simulink model "case7"  (R2024b)
settings: Solver=FixedStepAuto  StartTime=0  StopTime=1  FixedStep=1e-7  RelTol=1e-3
values from neighbouring files (symbols this model uses):
  SG_D_1_D = 0.01056    [IEEE9_case_parameters.m]    (also in case1_parameters.m; case2_parameters.m; case3_parameters.m; case4_parameters.m)
  SG_D_1_EnableSaturation = 0    [IEEE9_case_parameters.m]    (also in case1_parameters.m; case2_parameters.m; case3_parameters.m; case4_parameters.m)
  SG_D_1_f0 = 60    [IEEE9_case_parameters.m]    (also in case1_parameters.m; case2_parameters.m; case3_parameters.m; case4_parameters.m)
  SG_D_1_H = 7.5    [IEEE9_case_parameters.m]    (also in case1_parameters.m; case2_parameters.m; case3_parameters.m; case4_parameters.m)
  SG_D_1_K_A = 20    [IEEE9_case_parameters.m]    (also in case1_parameters.m; case2_parameters.m; case3_parameters.m; case4_parameters.m)
  SG_D_1_K_E = 1.000000e+1    (= 10)    [IEEE9_case_parameters.m]    (also in case1_parameters.m; case2_parameters.m; case3_parameters.m; case4_parameters.m)
  SG_D_1_K_F = 2.363    [IEEE9_case_parameters.m]    (also in case1_parameters.m; case2_parameters.m; case3_parameters.m; case4_parameters.m)
  SG_D_1_K_s = 0.5    [IEEE9_case_parameters.m]    (also in case1_parameters.m = 5; case2_parameters.m = 5; case3_parameters.m = 5; case4_parameters.m = 5)
  SG_D_1_R_a = 0.001088    [IEEE9_case_parameters.m]    (also in case1_parameters.m; case2_parameters.m; case3_parameters.m; case4_parameters.m)
  SG_D_1_S_A = 1    [IEEE9_case_parameters.m]    (also in case1_parameters.m; case2_parameters.m; case3_parameters.m; case4_parameters.m)
  SG_D_1_S_B = 0.103    [IEEE9_case_parameters.m]    (also in case1_parameters.m; case2_parameters.m; case3_parameters.m; case4_parameters.m)
  SG_D_1_S_N = 10.659857    [IEEE9_case_parameters.m]    (also in case1_parameters.m; case2_parameters.m; case3_parameters.m; case4_parameters.m)
  SG_D_1_SpeedPara = 200    [IEEE9_case_parameters.m]    (also in case1_parameters.m; case2_parameters.m; case3_parameters.m; case4_parameters.m)
  SG_D_1_T_0 = 0.720173    [IEEE9_case_parameters.m]    (also in case1_parameters.m = 0.755522; case2_parameters.m = 0.808931; case3_parameters.m = 0.869402; case4_parameters.m = 0.729316)
  SG_D_1_T_1 = 0.3    [IEEE9_case_parameters.m]    (also in case1_parameters.m; case2_parameters.m; case3_parameters.m; case4_parameters.m)
  SG_D_1_T_2 = 0.05    [IEEE9_case_parameters.m]    (also in case1_parameters.m; case2_parameters.m; case3_parameters.m; case4_parameters.m)
  SG_D_1_T_3 = 0.02    [IEEE9_case_parameters.m]    (also in case1_parameters.m; case2_parameters.m; case3_parameters.m; case4_parameters.m)
  SG_D_1_T_4 = 0.005    [IEEE9_case_parameters.m]    (also in case1_parameters.m; case2_parameters.m; case3_parameters.m; case4_parameters.m)
  SG_D_1_T_A = 0.02    [IEEE9_case_parameters.m]    (also in case1_parameters.m; case2_parameters.m; case3_parameters.m; case4_parameters.m)
  SG_D_1_T_dd = 8.000000e+0    (= 8)    [IEEE9_case_parameters.m]    (also in case1_parameters.m; case2_parameters.m; case3_parameters.m; case4_parameters.m)
  SG_D_1_T_ddd = 0.04    [IEEE9_case_parameters.m]    (also in case1_parameters.m; case2_parameters.m; case3_parameters.m; case4_parameters.m)
  SG_D_1_T_E = 0.314    [IEEE9_case_parameters.m]    (also in case1_parameters.m; case2_parameters.m; case3_parameters.m; case4_parameters.m)
  SG_D_1_T_F = 0.35    [IEEE9_case_parameters.m]    (also in case1_parameters.m; case2_parameters.m; case3_parameters.m; case4_parameters.m)
  SG_D_1_T_qd = 0.8    [IEEE9_case_parameters.m]    (also in case1_parameters.m; case2_parameters.m; case3_parameters.m; case4_parameters.m)
  SG_D_1_T_qdd = 0.02    [IEEE9_case_parameters.m]    (also in case1_parameters.m; case2_parameters.m; case3_parameters.m; case4_parameters.m)
  SG_D_1_T_speed = 0.1    [IEEE9_case_parameters.m]    (also in case1_parameters.m = 200; case2_parameters.m = 200; case3_parameters.m = 200; case4_parameters.m = 200)
  SG_D_1_T_w = 0.5    [IEEE9_case_parameters.m]    (also in case1_parameters.m; case2_parameters.m; case3_parameters.m; case4_parameters.m)
  SG_D_1_V_ref = 1.990276    [IEEE9_case_parameters.m]    (also in case1_parameters.m = 2.042296; case2_parameters.m = 2.051388; case3_parameters.m = 2.089584; case4_parameters.m = 2.01845)
  SG_D_1_w_ref = 376.991118    [IEEE9_case_parameters.m]    (also in case1_parameters.m; case2_parameters.m; case3_parameters.m; case4_parameters.m)
  SG_D_1_wb = 6.000000e+1    (= 60)    [IEEE9_case_parameters.m]    (also in case1_parameters.m; case2_parameters.m; case3_parameters.m; case4_parameters.m)
  SG_D_1_x_d = 1.9    [IEEE9_case_parameters.m]    (also in case1_parameters.m; case2_parameters.m; case3_parameters.m; case4_parameters.m)
  SG_D_1_x_dd = 0.302    [IEEE9_case_parameters.m]    (also in case1_parameters.m; case2_parameters.m; case3_parameters.m; case4_parameters.m)
  SG_D_1_x_ddd = 0.204    [IEEE9_case_parameters.m]    (also in case1_parameters.m; case2_parameters.m; case3_parameters.m; case4_parameters.m)
  SG_D_1_x_l = 0.05    [IEEE9_case_parameters.m]    (also in case1_parameters.m; case2_parameters.m; case3_parameters.m; case4_parameters.m)
  SG_D_1_x_q = 1.3    [IEEE9_case_parameters.m]    (also in case1_parameters.m; case2_parameters.m; case3_parameters.m; case4_parameters.m)
  SG_D_1_x_qd = 0.5    [IEEE9_case_parameters.m]    (also in case1_parameters.m; case2_parameters.m; case3_parameters.m; case4_parameters.m)
  SG_D_1_x_qdd = 0.3    [IEEE9_case_parameters.m]    (also in case1_parameters.m; case2_parameters.m; case3_parameters.m; case4_parameters.m)
  SG_D_2_D = 0.02    [IEEE9_case_parameters.m]    (also in case1_parameters.m; case2_parameters.m; case3_parameters.m; case4_parameters.m)
  SG_D_2_EnableSaturation = 0    [IEEE9_case_parameters.m]    (also in case1_parameters.m; case2_parameters.m; case3_parameters.m; case4_parameters.m)
  SG_D_2_f0 = 60    [IEEE9_case_parameters.m]    (also in case1_parameters.m; case2_parameters.m; case3_parameters.m; case4_parameters.m)
  SG_D_2_H = 8.000000e+0    (= 8)    [IEEE9_case_parameters.m]    (also in case1_parameters.m; case2_parameters.m; case3_parameters.m; case4_parameters.m)
  SG_D_2_K_A = 20    [IEEE9_case_parameters.m]    (also in case1_parameters.m; case2_parameters.m; case3_parameters.m; case4_parameters.m)
  SG_D_2_K_E = 1.000000e+1    (= 10)    [IEEE9_case_parameters.m]    (also in case1_parameters.m; case2_parameters.m; case3_parameters.m; case4_parameters.m)
  SG_D_2_K_F = 2.363    [IEEE9_case_parameters.m]    (also in case1_parameters.m; case2_parameters.m; case3_parameters.m; case4_parameters.m)
  SG_D_2_K_s = 0.5    [IEEE9_case_parameters.m]    (also in case1_parameters.m = 4; case2_parameters.m = 4; case3_parameters.m = 4; case4_parameters.m = 4)
  SG_D_2_R_a = 0.001088    [IEEE9_case_parameters.m]    (also in case1_parameters.m; case2_parameters.m; case3_parameters.m; case4_parameters.m)
  SG_D_2_S_A = 1    [IEEE9_case_parameters.m]    (also in case1_parameters.m; case2_parameters.m; case3_parameters.m; case4_parameters.m)
  SG_D_2_S_B = 0.103    [IEEE9_case_parameters.m]    (also in case1_parameters.m; case2_parameters.m; case3_parameters.m; case4_parameters.m)
  SG_D_2_S_N = 10.659857    [IEEE9_case_parameters.m]    (also in case1_parameters.m; case2_parameters.m; case3_parameters.m; case4_parameters.m)
  SG_D_2_SpeedPara = 200    [IEEE9_case_parameters.m]    (also in case1_parameters.m; case2_parameters.m; case3_parameters.m; case4_parameters.m)
  SG_D_2_T_0 = 1.632913    [IEEE9_case_parameters.m]    (also in case1_parameters.m = 1.632925; case2_parameters.m = 1.632915; case3_parameters.m = 1.632914; case4_parameters.m = 1.632927)
  SG_D_2_T_1 = 0.2    [IEEE9_case_parameters.m]    (also in case1_parameters.m; case2_parameters.m; case3_parameters.m; case4_parameters.m)
  SG_D_2_T_2 = 0.05    [IEEE9_case_parameters.m]    (also in case1_parameters.m; case2_parameters.m; case3_parameters.m; case4_parameters.m)
  SG_D_2_T_3 = 0.02    [IEEE9_case_parameters.m]    (also in case1_parameters.m; case2_parameters.m; case3_parameters.m; case4_parameters.m)
  SG_D_2_T_4 = 0.005    [IEEE9_case_parameters.m]    (also in case1_parameters.m; case2_parameters.m; case3_parameters.m; case4_parameters.m)
  SG_D_2_T_A = 0.02    [IEEE9_case_parameters.m]    (also in case1_parameters.m; case2_parameters.m; case3_parameters.m; case4_parameters.m)
  SG_D_2_T_dd = 7.9    [IEEE9_case_parameters.m]    (also in case1_parameters.m; case2_parameters.m; case3_parameters.m; case4_parameters.m)
  SG_D_2_T_ddd = 0.04    [IEEE9_case_parameters.m]    (also in case1_parameters.m; case2_parameters.m; case3_parameters.m; case4_parameters.m)
  SG_D_2_T_E = 0.314    [IEEE9_case_parameters.m]    (also in case1_parameters.m; case2_parameters.m; case3_parameters.m; case4_parameters.m)
  SG_D_2_T_F = 0.35    [IEEE9_case_parameters.m]    (also in case1_parameters.m; case2_parameters.m; case3_parameters.m; case4_parameters.m)
  SG_D_2_T_qd = 0.8    [IEEE9_case_parameters.m]    (also in case1_parameters.m; case2_parameters.m; case3_parameters.m; case4_parameters.m)
  SG_D_2_T_qdd = 0.015    [IEEE9_case_parameters.m]    (also in case1_parameters.m; case2_parameters.m; case3_parameters.m; case4_parameters.m)
  SG_D_2_T_speed = 0.1    [IEEE9_case_parameters.m]    (also in case1_parameters.m = 150; case2_parameters.m = 150; case3_parameters.m = 150; case4_parameters.m = 150)
  SG_D_2_T_w = 0.35    [IEEE9_case_parameters.m]    (also in case1_parameters.m; case2_parameters.m; case3_parameters.m; case4_parameters.m)
  SG_D_2_V_ref = 2.58547    [IEEE9_case_parameters.m]    (also in case1_parameters.m = 2.597896; case2_parameters.m = 2.587136; case3_parameters.m = 2.586042; case4_parameters.m = 2.599679)
  SG_D_2_w_ref = 376.991118    [IEEE9_case_parameters.m]    (also in case1_parameters.m; case2_parameters.m; case3_parameters.m; case4_parameters.m)
  SG_D_2_wb = 6.000000e+1    (= 60)    [IEEE9_case_parameters.m]    (also in case1_parameters.m; case2_parameters.m; case3_parameters.m; case4_parameters.m)
  SG_D_2_x_d = 1.8    [IEEE9_case_parameters.m]    (also in case1_parameters.m; case2_parameters.m; case3_parameters.m; case4_parameters.m)
  SG_D_2_x_dd = 0.302    [IEEE9_case_parameters.m]    (also in case1_parameters.m; case2_parameters.m; case3_parameters.m; case4_parameters.m)
  SG_D_2_x_ddd = 0.204    [IEEE9_case_parameters.m]    (also in case1_parameters.m; case2_parameters.m; case3_parameters.m; case4_parameters.m)
  SG_D_2_x_l = 0.05    [IEEE9_case_parameters.m]    (also in case1_parameters.m; case2_parameters.m; case3_parameters.m; case4_parameters.m)
  SG_D_2_x_q = 1.25    [IEEE9_case_parameters.m]    (also in case1_parameters.m; case2_parameters.m; case3_parameters.m; case4_parameters.m)
  SG_D_2_x_qd = 0.5    [IEEE9_case_parameters.m]    (also in case1_parameters.m; case2_parameters.m; case3_parameters.m; case4_parameters.m)
  SG_D_2_x_qdd = 0.3    [IEEE9_case_parameters.m]    (also in case1_parameters.m; case2_parameters.m; case3_parameters.m; case4_parameters.m)
  SG_D_3_D = 0.02    [IEEE9_case_parameters.m]    (also in case1_parameters.m; case2_parameters.m; case3_parameters.m; case4_parameters.m)
  SG_D_3_EnableSaturation = 0    [IEEE9_case_parameters.m]    (also in case1_parameters.m; case2_parameters.m; case3_parameters.m; case4_parameters.m)
  SG_D_3_f0 = 60    [IEEE9_case_parameters.m]    (also in case1_parameters.m; case2_parameters.m; case3_parameters.m; case4_parameters.m)
  SG_D_3_H = 7.7    [IEEE9_case_parameters.m]    (also in case1_parameters.m; case2_parameters.m; case3_parameters.m; case4_parameters.m)
  SG_D_3_K_A = 20    [IEEE9_case_parameters.m]    (also in case1_parameters.m; case2_parameters.m; case3_parameters.m; case4_parameters.m)
  SG_D_3_K_E = 1.000000e+1    (= 10)    [IEEE9_case_parameters.m]    (also in case1_parameters.m; case2_parameters.m; case3_parameters.m; case4_parameters.m)
  SG_D_3_K_F = 2.363    [IEEE9_case_parameters.m]    (also in case1_parameters.m; case2_parameters.m; case3_parameters.m; case4_parameters.m)
  SG_D_3_K_s = 0.2    [IEEE9_case_parameters.m]    (also in case1_parameters.m = 2; case2_parameters.m = 2; case3_parameters.m = 2; case4_parameters.m = 2)
  SG_D_3_R_a = 0.001088    [IEEE9_case_parameters.m]    (also in case1_parameters.m; case2_parameters.m; case3_parameters.m; case4_parameters.m)
  SG_D_3_S_A = 1    [IEEE9_case_parameters.m]    (also in case1_parameters.m; case2_parameters.m; case3_parameters.m; case4_parameters.m)
  SG_D_3_S_B = 0.103    [IEEE9_case_parameters.m]    (also in case1_parameters.m; case2_parameters.m; case3_parameters.m; case4_parameters.m)
  SG_D_3_S_N = 10.659857    [IEEE9_case_parameters.m]    (also in case1_parameters.m; case2_parameters.m; case3_parameters.m; case4_parameters.m)
  SG_D_3_SpeedPara = 200    [IEEE9_case_parameters.m]    (also in case1_parameters.m; case2_parameters.m; case3_parameters.m; case4_parameters.m)
  SG_D_3_T_0 = 0.850788    [IEEE9_case_parameters.m]    (also in case1_parameters.m = 0.850786; case2_parameters.m = 0.850787; case3_parameters.m; case4_parameters.m = 0.850786)
  SG_D_3_T_1 = 0.2    [IEEE9_case_parameters.m]    (also in case1_parameters.m; case2_parameters.m; case3_parameters.m; case4_parameters.m)
  SG_D_3_T_2 = 0.05    [IEEE9_case_parameters.m]    (also in case1_parameters.m; case2_parameters.m; case3_parameters.m; case4_parameters.m)
  SG_D_3_T_3 = 0.02    [IEEE9_case_parameters.m]    (also in case1_parameters.m; case2_parameters.m; case3_parameters.m; case4_parameters.m)
  SG_D_3_T_4 = 0.005    [IEEE9_case_parameters.m]    (also in case1_parameters.m; case2_parameters.m; case3_parameters.m; case4_parameters.m)
  SG_D_3_T_A = 0.02    [IEEE9_case_parameters.m]    (also in case1_parameters.m; case2_parameters.m; case3_parameters.m; case4_parameters.m)
  SG_D_3_T_dd = 8.1    [IEEE9_case_parameters.m]    (also in case1_parameters.m; case2_parameters.m; case3_parameters.m; case4_parameters.m)
  SG_D_3_T_ddd = 0.04    [IEEE9_case_parameters.m]    (also in case1_parameters.m; case2_parameters.m; case3_parameters.m; case4_parameters.m)
  SG_D_3_T_E = 0.314    [IEEE9_case_parameters.m]    (also in case1_parameters.m; case2_parameters.m; case3_parameters.m; case4_parameters.m)
  SG_D_3_T_F = 0.35    [IEEE9_case_parameters.m]    (also in case1_parameters.m; case2_parameters.m; case3_parameters.m; case4_parameters.m)
  SG_D_3_T_qd = 0.8    [IEEE9_case_parameters.m]    (also in case1_parameters.m; case2_parameters.m; case3_parameters.m; case4_parameters.m)
  SG_D_3_T_qdd = 0.015    [IEEE9_case_parameters.m]    (also in case1_parameters.m; case2_parameters.m; case3_parameters.m; case4_parameters.m)
  SG_D_3_T_speed = 0.1    [IEEE9_case_parameters.m]    (also in case1_parameters.m = 180; case2_parameters.m = 180; case3_parameters.m = 180; case4_parameters.m = 180)
  SG_D_3_T_w = 0.4    [IEEE9_case_parameters.m]    (also in case1_parameters.m; case2_parameters.m; case3_parameters.m; case4_parameters.m)
  SG_D_3_V_ref = 1.892727    [IEEE9_case_parameters.m]    (also in case1_parameters.m = 1.906439; case2_parameters.m = 1.895535; case3_parameters.m = 1.892105; case4_parameters.m = 1.906598)
  SG_D_3_w_ref = 376.991118    [IEEE9_case_parameters.m]    (also in case1_parameters.m; case2_parameters.m; case3_parameters.m; case4_parameters.m)
  SG_D_3_wb = 6.000000e+1    (= 60)    [IEEE9_case_parameters.m]    (also in case1_parameters.m; case2_parameters.m; case3_parameters.m; case4_parameters.m)
  SG_D_3_x_d = 1.85    [IEEE9_case_parameters.m]    (also in case1_parameters.m; case2_parameters.m; case3_parameters.m; case4_parameters.m)
  SG_D_3_x_dd = 0.302    [IEEE9_case_parameters.m]    (also in case1_parameters.m; case2_parameters.m; case3_parameters.m; case4_parameters.m)
  SG_D_3_x_ddd = 0.204    [IEEE9_case_parameters.m]    (also in case1_parameters.m; case2_parameters.m; case3_parameters.m; case4_parameters.m)
  SG_D_3_x_l = 0.05    [IEEE9_case_parameters.m]    (also in case1_parameters.m; case2_parameters.m; case3_parameters.m; case4_parameters.m)
  SG_D_3_x_q = 1.2    [IEEE9_case_parameters.m]    (also in case1_parameters.m; case2_parameters.m; case3_parameters.m; case4_parameters.m)
  SG_D_3_x_qd = 0.5    [IEEE9_case_parameters.m]    (also in case1_parameters.m; case2_parameters.m; case3_parameters.m; case4_parameters.m)
  SG_D_3_x_qdd = 0.3    [IEEE9_case_parameters.m]    (also in case1_parameters.m; case2_parameters.m; case3_parameters.m; case4_parameters.m)
(part 5 of 12)

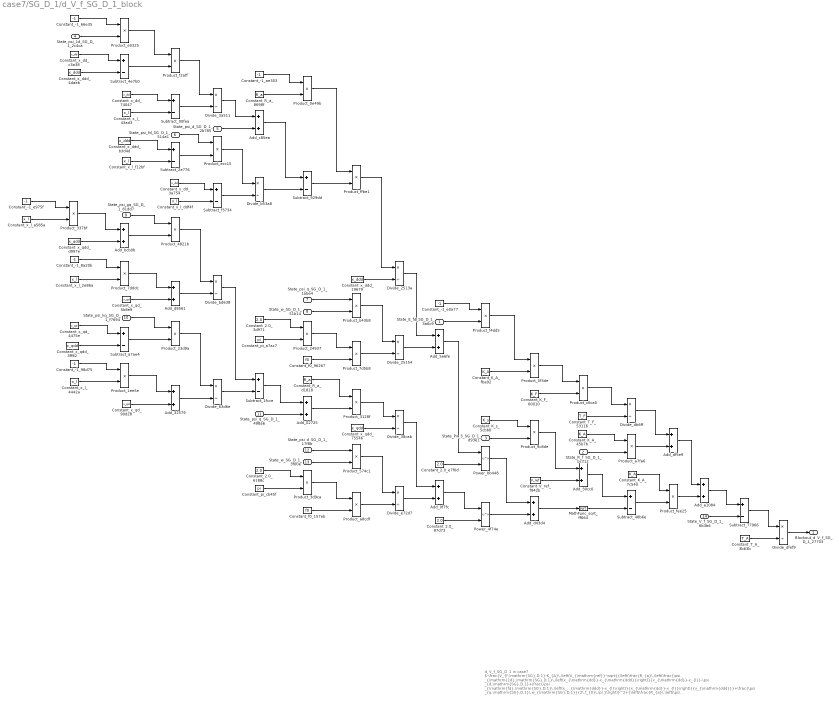
== system case7/SG_D_1/d_V_f_SG_D_1_block ==
  note: d_V_f_SG_D_1 in case7
      | $-\frac{V_{f,\mathrm{SG},D,1}-K_{A}\,\left(V_{\mathrm{ref}}-\sqrt{{\left(\frac{R_{a}\,\left(\frac{\psi _{\mathrm{1d},\mathrm{SG},D,1}\,\left(x_{\mathrm{dd}}-x_{\mathrm{ddd}}\right)}{x_{\mathrm{dd}}-x_{l}}-\psi _{d,\mathrm{SG},D,1}+\frac{\psi _{\mathrm{fd},\mathrm{SG},D,1}\,\left(x_{\mathrm{ddd}}-x_{l}\right)}{x_{\mathrm{dd}}-x_{l}}\right)}{x_{\mathrm{ddd}}}+\frac{\psi _{q,\mathrm{SG},D,1}\,w_{\mathrm{SG},D,1}}{2\,f_{0}\,\pi }\right)}^2+{\left(\frac{R_{a}\,\left(\psi _{q,\mathrm{SG},D,1}+\frac{\psi _{\mathrm{gq},\mathrm{SG},D,1}\,\left(x_{l}-x_{\mathrm{qdd}}\right)}{x_{l}-x_{\mathrm{qd}}}+\frac{\psi _{\mathrm{kq},\mathrm{SG},D,1}\,\left(x_{\mathrm{qd}}-x_{\mathrm{qdd}}\right)}{x_{l}-x_{\mathrm{qd}}}\right)}{x_{\mathrm{qdd}}}+\frac{\psi _{d,\mathrm{SG},D,1}\,w_{\mathrm{SG},D,1}}{2\,f_{0}\,\pi }\right)}^2}+K_{s}\,\mathrm{Px}_{3,\mathrm{SG},D,1}\right)-K_{A}\,R_{f,\mathrm{SG},D,1}+\frac{E_{\mathrm{fd},\mathrm{SG},D,1}\,K_{A}\,K_{F}}{T_{F}}}{T_{A}}$
      | Automatically generated on 2025-10-31 19:23:40 .
  State_E_fd_SG_D_1_3a6c9 : Inport
  State_R_f_SG_D_1_bc712 : Inport  Port=2
  State_Px_3_SG_D_1_d93e1 : Inport  Port=3
  State_psi_1d_SG_D_1_2c4ca : Inport  Port=4
  State_psi_d_SG_D_1_2b785 : Inport  Port=5
  State_psi_fd_SG_D_1_514a1 : Inport  Port=6
  State_psi_q_SG_D_1_1abe4 : Inport  Port=7
  State_w_SG_D_1_51b14 : Inport  Port=8
  State_psi_gq_SG_D_1_81dd7 : Inport  Port=9
  State_psi_kq_SG_D_1_f7694 : Inport  Port=10
  State_psi_q_SG_D_1_498a6 : Inport  Port=11
  State_psi_d_SG_D_1_17f8b : Inport  Port=12
  State_w_SG_D_1_3f00e : Inport  Port=13
  State_V_f_SG_D_1_6b3b6 : Inport  Port=14
  Add_02725 : Sum
  Add_0f7fc : Sum
  Add_30cc0 : Sum
  Add_32579 : Sum
  Add_5e6fe : Sum
  Add_a1084 : Sum
  Add_bcb0b : Sum
  Add_c85ea : Sum
  Add_d43d4 : Sum
  Add_d8561 : Sum
  Add_df5e9 : Sum
  Constant_-1_66e35 : Constant  Value=-1
  Constant_-1_8a20b : Constant  Value=-1
  Constant_-1_98d75 : Constant  Value=-1
  Constant_-1_ae303 : Constant  Value=-1
  Constant_-1_e0a77 : Constant  Value=-1
  Constant_-1_e975f : Constant  Value=-1
  Constant_2.0_3d971 : Constant  Value=2.0
  Constant_2.0_6188c : Constant  Value=2.0
  Constant_2.0_87d73 : Constant  Value=2.0
  Constant_2.0_e7f0d : Constant  Value=2.0
  Constant_K_A_45b7b : Constant  Value=K_A
  Constant_K_A_7c54d : Constant  Value=K_A
  Constant_K_A_fba92 : Constant  Value=K_A
  Constant_K_F_60010 : Constant  Value=K_F
  Constant_K_s_5cbbb : Constant  Value=K_s
  Constant_R_a_8698f : Constant  Value=R_a
  Constant_R_a_d1818 : Constant  Value=R_a
  Constant_T_A_3b63b : Constant  Value=T_A
  Constant_T_F_53116 : Constant  Value=T_F
  Constant_V_ref_f942b : Constant  Value=V_ref
  Constant_f0_157eb : Constant  Value=f0
  Constant_f0_96267 : Constant  Value=f0
  Constant_pi_a7ac7 : Constant  Value=pi
  Constant_pi_cb45f : Constant  Value=pi
  Constant_x_dd_3a754 : Constant  Value=x_dd
  Constant_x_dd_74047 : Constant  Value=x_dd
  Constant_x_dd_c3a38 : Constant  Value=x_dd
  Constant_x_ddd_19679 : Constant  Value=x_ddd
  Constant_x_ddd_4daeb : Constant  Value=x_ddd
  Constant_x_ddd_b3d4d : Constant  Value=x_ddd
  Constant_x_l_2e86a : Constant  Value=x_l
  Constant_x_l_43ad3 : Constant  Value=x_l
  Constant_x_l_4442a : Constant  Value=x_l
  Constant_x_l_a585a : Constant  Value=x_l
  Constant_x_l_ddf4f : Constant  Value=x_l
  Constant_x_l_f12bf : Constant  Value=x_l
  Constant_x_qd_4475e : Constant  Value=x_qd
  Constant_x_qd_5b8e9 : Constant  Value=x_qd
  Constant_x_qd_90d28 : Constant  Value=x_qd
  Constant_x_qdd_3ff82 : Constant  Value=x_qdd
  Constant_x_qdd_75546 : Constant  Value=x_qdd
  Constant_x_qdd_d997e : Constant  Value=x_qdd
  Divide_2513a : Product  Inputs=*/
  Divide_25154 : Product  Inputs=*/
  Divide_38cab : Product  Inputs=*/
  Divide_3a511 : Product  Inputs=*/
  Divide_63d6e : Product  Inputs=*/
  Divide_b53a8 : Product  Inputs=*/
  Divide_bd638 : Product  Inputs=*/
  Divide_db6ff : Product  Inputs=*/
  Divide_dfef9 : Product  Inputs=*/
  Divide_e72d7 : Product  Inputs=*/
  MathFunc_sqrt_ff664 : Sqrt
  Power_4f74e : Math  Operator=pow
  Power_bb448 : Math  Operator=pow
  Product_0e49b : Product
  Product_1ee5e : Product
  Product_23d9a : Product
  Product_24937 : Product
  Product_3128f : Product
  Product_337bf : Product
  Product_3d9ca : Product
  Product_4821b : Product
  Product_574c1 : Product
  Product_5f3de : Product
  Product_7d5b8 : Product
  Product_7dddc : Product
  Product_9c8de : Product
  Product_a7fa6 : Product
  Product_a8cdf : Product
  Product_b43b8 : Product
  Product_c6ca0 : Product
  Product_e0325 : Product
  Product_ecc15 : Product
  Product_f2aff : Product
  Product_f4dd5 : Product
  Product_fee25 : Product
  Product_ffbe1 : Product
  Subtract_00fea : Sum  Inputs=+-
  Subtract_1fcce : Sum  Inputs=+-
  Subtract_2e776 : Sum  Inputs=+-
  Subtract_48b6e : Sum  Inputs=+-
  Subtract_4e7b0 : Sum  Inputs=+-
  Subtract_77966 : Sum  Inputs=+-
  Subtract_929dd : Sum  Inputs=+-
  Subtract_a7ae4 : Sum  Inputs=+-
  Subtract_f3734 : Sum  Inputs=+-
  Blockout_d_V_f_SG_D_1_27703 : Outport
  wires:
  Constant_-1_98d75/1 -> Product_1ee5e/1
  Constant_-1_e975f/1 -> Product_337bf/1
  State_psi_d_SG_D_1_17f8b/1 -> Product_574c1/1
  Constant_x_qd_90d28/1 -> Add_32579/2
  Constant_x_qdd_d997e/1 -> Add_bcb0b/2
  State_w_SG_D_1_3f00e/1 -> Product_574c1/2
  Constant_x_l_a585a/1 -> Product_337bf/2
  Subtract_929dd/1 -> Product_ffbe1/2
  Constant_x_l_4442a/1 -> Product_1ee5e/2
  Constant_x_dd_c3a38/1 -> Subtract_4e7b0/1
  Constant_R_a_8698f/1 -> Product_0e49b/2
  Constant_-1_66e35/1 -> Product_e0325/1
  Divide_b53a8/1 -> Subtract_929dd/2
  Constant_x_ddd_4daeb/1 -> Subtract_4e7b0/2
  Add_32579/1 -> Divide_63d6e/2
  State_psi_1d_SG_D_1_2c4ca/1 -> Product_e0325/2
  Add_d8561/1 -> Divide_bd638/2
  Subtract_a7ae4/1 -> Product_23d9a/2
  Product_c6ca0/1 -> Divide_db6ff/1
  Product_24937/1 -> Product_7d5b8/1
  Product_337bf/1 -> Add_bcb0b/1
  Constant_-1_8a20b/1 -> Product_7dddc/1
  Constant_x_l_2e86a/1 -> Product_7dddc/2
  Add_c85ea/1 -> Subtract_929dd/1
  Constant_2.0_6188c/1 -> Product_3d9ca/1
  Constant_x_qd_4475e/1 -> Subtract_a7ae4/1
  Product_e0325/1 -> Product_f2aff/1
  Constant_pi_cb45f/1 -> Product_3d9ca/2
  Constant_x_qdd_3ff82/1 -> Subtract_a7ae4/2
  Subtract_4e7b0/1 -> Product_f2aff/2
  State_psi_q_SG_D_1_498a6/1 -> Add_02725/2
  Constant_x_dd_74047/1 -> Subtract_00fea/1
  Constant_x_l_43ad3/1 -> Subtract_00fea/2
  Constant_x_ddd_b3d4d/1 -> Subtract_2e776/1
  Constant_x_l_f12bf/1 -> Subtract_2e776/2
  State_psi_gq_SG_D_1_81dd7/1 -> Product_4821b/1
  Add_bcb0b/1 -> Product_4821b/2
  Product_7dddc/1 -> Add_d8561/1
  Constant_x_qd_5b8e9/1 -> Add_d8561/2
  Divide_3a511/1 -> Add_c85ea/1
  Subtract_00fea/1 -> Divide_3a511/2
  State_psi_kq_SG_D_1_f7694/1 -> Product_23d9a/1
  Divide_dfef9/1 -> Blockout_d_V_f_SG_D_1_27703/1
  Product_1ee5e/1 -> Add_32579/1
  Product_f2aff/1 -> Divide_3a511/1
  State_psi_fd_SG_D_1_514a1/1 -> Product_ecc15/1
  State_w_SG_D_1_51b14/1 -> Product_b43b8/2
  Subtract_2e776/1 -> Product_ecc15/2
  Constant_x_dd_3a754/1 -> Subtract_f3734/1
  Constant_x_l_ddf4f/1 -> Subtract_f3734/2
  Product_4821b/1 -> Divide_bd638/1
  Product_0e49b/1 -> Product_ffbe1/1
  Product_23d9a/1 -> Divide_63d6e/1
  State_psi_d_SG_D_1_2b785/1 -> Add_c85ea/2
  Product_ecc15/1 -> Divide_b53a8/1
  Subtract_f3734/1 -> Divide_b53a8/2
  Divide_bd638/1 -> Subtract_1fcce/1
  Divide_63d6e/1 -> Subtract_1fcce/2
  Constant_-1_ae303/1 -> Product_0e49b/1
  Constant_2.0_3d971/1 -> Product_24937/1
  Constant_pi_a7ac7/1 -> Product_24937/2
  Subtract_1fcce/1 -> Add_02725/1
  State_psi_q_SG_D_1_1abe4/1 -> Product_b43b8/1
  Constant_f0_96267/1 -> Product_7d5b8/2
  Constant_R_a_d1818/1 -> Product_3128f/1
  Add_02725/1 -> Product_3128f/2
  Product_3d9ca/1 -> Product_a8cdf/1
  Power_bb448/1 -> Add_d43d4/1
  Constant_f0_157eb/1 -> Product_a8cdf/2
  Product_ffbe1/1 -> Divide_2513a/1
  Constant_x_ddd_19679/1 -> Divide_2513a/2
  Product_b43b8/1 -> Divide_25154/1
  Product_7d5b8/1 -> Divide_25154/2
  Product_3128f/1 -> Divide_38cab/1
  Constant_x_qdd_75546/1 -> Divide_38cab/2
  Product_574c1/1 -> Divide_e72d7/1
  Product_a8cdf/1 -> Divide_e72d7/2
  Divide_2513a/1 -> Add_5e6fe/1
  Divide_25154/1 -> Add_5e6fe/2
  Divide_38cab/1 -> Add_0f7fc/1
  Divide_e72d7/1 -> Add_0f7fc/2
  Constant_-1_e0a77/1 -> Product_f4dd5/1
  State_E_fd_SG_D_1_3a6c9/1 -> Product_f4dd5/2
  Add_5e6fe/1 -> Power_bb448/1
  Constant_2.0_e7f0d/1 -> Power_bb448/2
  Add_0f7fc/1 -> Power_4f74e/1
  Constant_2.0_87d73/1 -> Power_4f74e/2
  Product_f4dd5/1 -> Product_5f3de/1
  Constant_K_A_fba92/1 -> Product_5f3de/2
  Constant_K_s_5cbbb/1 -> Product_9c8de/1
  State_Px_3_SG_D_1_d93e1/1 -> Product_9c8de/2
  Power_4f74e/1 -> Add_d43d4/2
  Divide_db6ff/1 -> Add_df5e9/1
  Product_5f3de/1 -> Product_c6ca0/1
  Constant_K_F_60010/1 -> Product_c6ca0/2
  Product_9c8de/1 -> Add_30cc0/1
  Constant_V_ref_f942b/1 -> Add_30cc0/2
  Add_d43d4/1 -> MathFunc_sqrt_ff664/1
  Constant_T_F_53116/1 -> Divide_db6ff/2
  Constant_K_A_45b7b/1 -> Product_a7fa6/1
  State_R_f_SG_D_1_bc712/1 -> Product_a7fa6/2
  Add_30cc0/1 -> Subtract_48b6e/1
  MathFunc_sqrt_ff664/1 -> Subtract_48b6e/2
  Constant_T_A_3b63b/1 -> Divide_dfef9/2
  Product_a7fa6/1 -> Add_df5e9/2
  Constant_K_A_7c54d/1 -> Product_fee25/1
  Subtract_48b6e/1 -> Product_fee25/2
  Add_df5e9/1 -> Add_a1084/1
  Product_fee25/1 -> Add_a1084/2
  Add_a1084/1 -> Subtract_77966/1
  State_V_f_SG_D_1_6b3b6/1 -> Subtract_77966/2
  Subtract_77966/1 -> Divide_dfef9/1

== system case7/SG_D_1/d_psi_1d_SG_D_1_block ==
  note: d_psi_1d_SG_D_1 in case7
      | $-\frac{\psi _{\mathrm{1d},\mathrm{SG},D,1}-\psi _{\mathrm{fd},\mathrm{SG},D,1}+\frac{\left(x_{\mathrm{dd}}-x_{l}\right)\,\left(\frac{\psi _{\mathrm{1d},\mathrm{SG},D,1}\,\left(x_{\mathrm{dd}}-x_{\mathrm{ddd}}\right)}{x_{\mathrm{dd}}-x_{l}}-\psi _{d,\mathrm{SG},D,1}+\frac{\psi _{\mathrm{fd},\mathrm{SG},D,1}\,\left(x_{\mathrm{ddd}}-x_{l}\right)}{x_{\mathrm{dd}}-x_{l}}\right)}{x_{\mathrm{ddd}}}}{T_{\mathrm{ddd}}}$
      | Automatically generated on 2025-10-31 19:23:15 .
  State_psi_1d_SG_D_1_e7f45 : Inport
  State_psi_fd_SG_D_1_1ada6 : Inport  Port=2
  State_psi_1d_SG_D_1_ed62b : Inport  Port=3
  State_psi_d_SG_D_1_1ea7c : Inport  Port=4
  State_psi_fd_SG_D_1_e0875 : Inport  Port=5
  Add_3b064 : Sum
  Add_ae224 : Sum
  Add_bc5e9 : Sum
  Constant_-1_28f6b : Constant  Value=-1
  Constant_-1_75077 : Constant  Value=-1
  Constant_T_ddd_53307 : Constant  Value=T_ddd
  Constant_x_dd_2d2f8 : Constant  Value=x_dd
  Constant_x_dd_5160e : Constant  Value=x_dd
  Constant_x_dd_8c47e : Constant  Value=x_dd
  Constant_x_dd_fe7fc : Constant  Value=x_dd
  Constant_x_ddd_30575 : Constant  Value=x_ddd
  Constant_x_ddd_5055e : Constant  Value=x_ddd
  Constant_x_ddd_c35db : Constant  Value=x_ddd
  Constant_x_l_9b483 : Constant  Value=x_l
  Constant_x_l_ad5c1 : Constant  Value=x_l
  Constant_x_l_c8eb9 : Constant  Value=x_l
  Constant_x_l_e7cfa : Constant  Value=x_l
  Divide_7d39b : Product  Inputs=*/
  Divide_94cca : Product  Inputs=*/
  Divide_d1690 : Product  Inputs=*/
  Divide_f2441 : Product  Inputs=*/
  Product_2a93d : Product
  Product_5d386 : Product
  Product_a18b3 : Product
  Product_d6a1f : Product
  Product_d7ceb : Product
  Subtract_12fd5 : Sum  Inputs=+-
  Subtract_2a5ae : Sum  Inputs=+-
  Subtract_4fa28 : Sum  Inputs=+-
  Subtract_633df : Sum  Inputs=+-
  Subtract_920c5 : Sum  Inputs=+-
  Subtract_acd1f : Sum  Inputs=+-
  Blockout_d_psi_1d_SG_D_1_e2098 : Outport
  wires:
  Product_d6a1f/1 -> Product_a18b3/1
  Constant_-1_28f6b/1 -> Product_d6a1f/1
  Subtract_12fd5/1 -> Product_a18b3/2
  State_psi_1d_SG_D_1_ed62b/1 -> Product_d6a1f/2
  Subtract_633df/1 -> Product_d7ceb/1
  State_psi_d_SG_D_1_1ea7c/1 -> Add_bc5e9/2
  Constant_x_dd_8c47e/1 -> Subtract_4fa28/1
  Constant_x_l_9b483/1 -> Subtract_633df/2
  Constant_x_dd_5160e/1 -> Subtract_12fd5/1
  Subtract_2a5ae/1 -> Product_5d386/2
  Constant_x_l_ad5c1/1 -> Subtract_4fa28/2
  Divide_7d39b/1 -> Subtract_920c5/2
  Constant_x_ddd_30575/1 -> Subtract_12fd5/2
  Constant_x_ddd_5055e/1 -> Subtract_2a5ae/1
  Constant_x_l_c8eb9/1 -> Subtract_2a5ae/2
  Add_3b064/1 -> Add_ae224/1
  Product_a18b3/1 -> Divide_d1690/1
  Divide_f2441/1 -> Add_ae224/2
  Subtract_4fa28/1 -> Divide_d1690/2
  State_psi_fd_SG_D_1_e0875/1 -> Product_5d386/1
  Constant_x_dd_fe7fc/1 -> Subtract_acd1f/1
  Constant_x_l_e7cfa/1 -> Subtract_acd1f/2
  Constant_x_ddd_c35db/1 -> Divide_f2441/2
  Subtract_920c5/1 -> Product_d7ceb/2
  Divide_d1690/1 -> Add_bc5e9/1
  Product_5d386/1 -> Divide_7d39b/1
  Subtract_acd1f/1 -> Divide_7d39b/2
  Product_d7ceb/1 -> Divide_f2441/1
  Constant_x_dd_2d2f8/1 -> Subtract_633df/1
  Add_bc5e9/1 -> Subtract_920c5/1
  Constant_-1_75077/1 -> Product_2a93d/1
  State_psi_1d_SG_D_1_e7f45/1 -> Product_2a93d/2
  Product_2a93d/1 -> Add_3b064/1
  State_psi_fd_SG_D_1_1ada6/1 -> Add_3b064/2
  Add_ae224/1 -> Divide_94cca/1
  Constant_T_ddd_53307/1 -> Divide_94cca/2
  Divide_94cca/1 -> Blockout_d_psi_1d_SG_D_1_e2098/1

== system case7/SG_D_1/d_psi_d_SG_D_1_block ==
  note: d_psi_d_SG_D_1 in case7
      | $2\,\pi \,f_{0}\,\left(v_{d,\mathrm{SG},D,1}\,\sin\left(\theta _{\mathrm{SG},D,1}\right)-v_{q,\mathrm{SG},D,1}\,\cos\left(\theta _{\mathrm{SG},D,1}\right)+\frac{R_{a}\,\left(\frac{\psi _{\mathrm{1d},\mathrm{SG},D,1}\,\left(x_{\mathrm{dd}}-x_{\mathrm{ddd}}\right)}{x_{\mathrm{dd}}-x_{l}}-\psi _{d,\mathrm{SG},D,1}+\frac{\psi _{\mathrm{fd},\mathrm{SG},D,1}\,\left(x_{\mathrm{ddd}}-x_{l}\right)}{x_{\mathrm{dd}}-x_{l}}\right)}{x_{\mathrm{ddd}}}+\frac{\psi _{q,\mathrm{SG},D,1}\,w_{\mathrm{SG},D,1}}{2\,f_{0}\,\pi }\right)$
      | Automatically generated on 2025-10-31 19:22:49 .
  State_psi_1d_SG_D_1_721c9 : Inport
  State_psi_d_SG_D_1_516f9 : Inport  Port=2
  State_psi_fd_SG_D_1_b0bb2 : Inport  Port=3
  Input_v_d_SG_D_1_36932 : Inport  Port=4
  State_theta_SG_D_1_2d59f : Inport  Port=5
  Input_v_q_SG_D_1_29a14 : Inport  Port=6
  State_theta_SG_D_1_b3d69 : Inport  Port=7
  State_psi_q_SG_D_1_df331 : Inport  Port=8
  State_w_SG_D_1_d723e : Inport  Port=9
  Add_3ffff : Sum
  Add_cd59b : Sum
  Constant_-1_520aa : Constant  Value=-1
  Constant_-2.0_35b4f : Constant  Value=-2.0
  Constant_2.0_e2e08 : Constant  Value=2.0
  Constant_R_a_f5feb : Constant  Value=R_a
  Constant_f0_86f8f : Constant  Value=f0
  Constant_f0_f0211 : Constant  Value=f0
  Constant_pi_10833 : Constant  Value=pi
  Constant_pi_dd50f : Constant  Value=pi
  Constant_x_dd_1f9cc : Constant  Value=x_dd
  Constant_x_dd_23065 : Constant  Value=x_dd
  Constant_x_dd_dbd8f : Constant  Value=x_dd
  Constant_x_ddd_39e1c : Constant  Value=x_ddd
  Constant_x_ddd_40f01 : Constant  Value=x_ddd
  Constant_x_ddd_b9199 : Constant  Value=x_ddd
  Constant_x_l_1b566 : Constant  Value=x_l
  Constant_x_l_8c137 : Constant  Value=x_l
  Constant_x_l_bc0ba : Constant  Value=x_l
  Divide_2b96e : Product  Inputs=*/
  Divide_72fe4 : Product  Inputs=*/
  Divide_7a059 : Product  Inputs=*/
  Divide_8d1e4 : Product  Inputs=*/
  MathFunc_cos_9b608 : Trigonometry  Operator=cos
  MathFunc_sin_e15c4 : Trigonometry
  Product_18dd6 : Product
  Product_1e699 : Product
  Product_2363c : Product
  Product_33f97 : Product
  Product_3a328 : Product
  Product_427e1 : Product
  Product_54e2f : Product
  Product_78055 : Product
  Product_9693d : Product
  Product_c79a8 : Product
  Product_da1b4 : Product
  Product_dd05b : Product
  Subtract_11176 : Sum  Inputs=+-
  Subtract_7c284 : Sum  Inputs=+-
  Subtract_ac3fe : Sum  Inputs=+-
  Subtract_c517e : Sum  Inputs=+-
  Subtract_e7ecc : Sum  Inputs=+-
  Subtract_f5d44 : Sum  Inputs=+-
  Subtract_fdbba : Sum  Inputs=+-
  Blockout_d_psi_d_SG_D_1_499f8 : Outport
  wires:
  Add_cd59b/1 -> Subtract_11176/1
  Product_54e2f/1 -> Divide_72fe4/1
  Subtract_e7ecc/1 -> Product_54e2f/2
  Divide_72fe4/1 -> Add_cd59b/1
  Product_18dd6/1 -> Product_54e2f/1
  Constant_x_ddd_39e1c/1 -> Subtract_e7ecc/2
  Constant_x_dd_23065/1 -> Subtract_e7ecc/1
  State_psi_1d_SG_D_1_721c9/1 -> Product_18dd6/2
  Constant_-1_520aa/1 -> Product_18dd6/1
  Product_dd05b/1 -> Divide_7a059/1
  Constant_x_l_1b566/1 -> Subtract_fdbba/2
  State_psi_d_SG_D_1_516f9/1 -> Add_cd59b/2
  Constant_x_dd_1f9cc/1 -> Subtract_fdbba/1
  Constant_x_ddd_40f01/1 -> Subtract_7c284/1
  Constant_x_l_8c137/1 -> Subtract_7c284/2
  Subtract_fdbba/1 -> Divide_72fe4/2
  State_psi_fd_SG_D_1_b0bb2/1 -> Product_dd05b/1
  Constant_x_ddd_b9199/1 -> Divide_2b96e/2
  Subtract_7c284/1 -> Product_dd05b/2
  Product_9693d/1 -> Subtract_c517e/2
  Constant_x_dd_dbd8f/1 -> Subtract_f5d44/1
  Constant_x_l_bc0ba/1 -> Subtract_f5d44/2
  Subtract_f5d44/1 -> Divide_7a059/2
  Divide_7a059/1 -> Subtract_11176/2
  Constant_R_a_f5feb/1 -> Product_33f97/1
  Subtract_11176/1 -> Product_33f97/2
  MathFunc_cos_9b608/1 -> Product_2363c/2
  State_theta_SG_D_1_2d59f/1 -> MathFunc_sin_e15c4/1
  Divide_2b96e/1 -> Subtract_c517e/1
  Product_33f97/1 -> Divide_2b96e/1
  MathFunc_sin_e15c4/1 -> Product_9693d/2
  Input_v_d_SG_D_1_36932/1 -> Product_9693d/1
  Product_c79a8/1 -> Blockout_d_psi_d_SG_D_1_499f8/1
  Product_da1b4/1 -> Product_c79a8/1
  Product_3a328/1 -> Product_da1b4/1
  State_theta_SG_D_1_b3d69/1 -> MathFunc_cos_9b608/1
  Constant_2.0_e2e08/1 -> Product_427e1/1
  Constant_pi_dd50f/1 -> Product_427e1/2
  Input_v_q_SG_D_1_29a14/1 -> Product_2363c/1
  Constant_f0_f0211/1 -> Product_da1b4/2
  State_psi_q_SG_D_1_df331/1 -> Product_78055/1
  State_w_SG_D_1_d723e/1 -> Product_78055/2
  Product_427e1/1 -> Product_1e699/1
  Constant_pi_10833/1 -> Product_3a328/2
  Constant_f0_86f8f/1 -> Product_1e699/2
  Constant_-2.0_35b4f/1 -> Product_3a328/1
  Add_3ffff/1 -> Subtract_ac3fe/1
  Subtract_c517e/1 -> Add_3ffff/1
  Product_2363c/1 -> Add_3ffff/2
  Product_78055/1 -> Divide_8d1e4/1
  Product_1e699/1 -> Divide_8d1e4/2
  Divide_8d1e4/1 -> Subtract_ac3fe/2
  Subtract_ac3fe/1 -> Product_c79a8/2

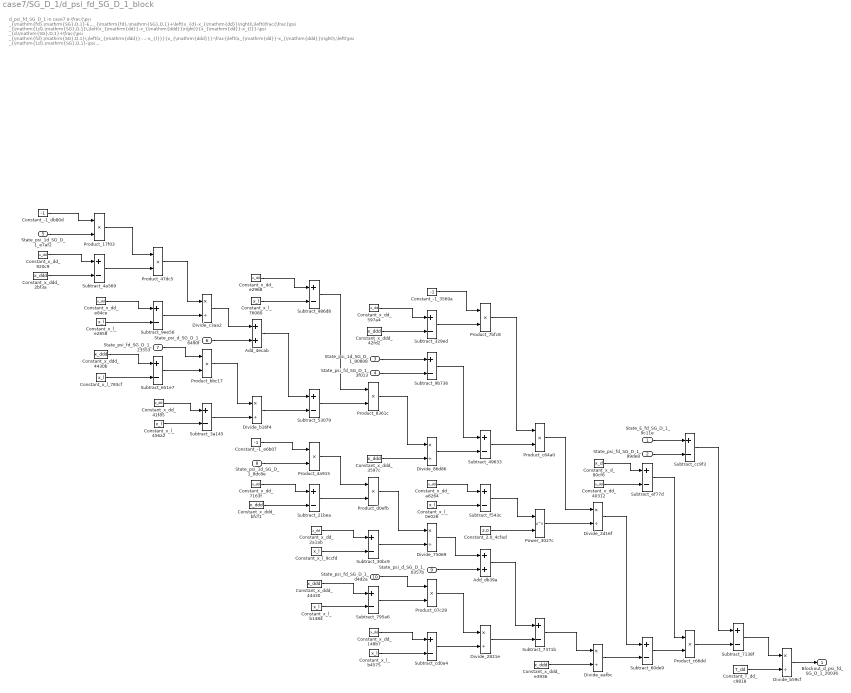
== system case7/SG_D_1/d_psi_fd_SG_D_1_block ==
  note: d_psi_fd_SG_D_1 in case7
      | $-\frac{\psi _{\mathrm{fd},\mathrm{SG},D,1}-E_{\mathrm{fd},\mathrm{SG},D,1}+\left(x_{d}-x_{\mathrm{dd}}\right)\,\left(\frac{\frac{\psi _{\mathrm{1d},\mathrm{SG},D,1}\,\left(x_{\mathrm{dd}}-x_{\mathrm{ddd}}\right)}{x_{\mathrm{dd}}-x_{l}}-\psi _{d,\mathrm{SG},D,1}+\frac{\psi _{\mathrm{fd},\mathrm{SG},D,1}\,\left(x_{\mathrm{ddd}}-x_{l}\right)}{x_{\mathrm{dd}}-x_{l}}}{x_{\mathrm{ddd}}}-\frac{\left(x_{\mathrm{dd}}-x_{\mathrm{ddd}}\right)\,\left(\psi _{\mathrm{1d},\mathrm{SG},D,1}-\psi _{\mathrm{fd},\mathrm{SG},D,1}+\frac{\left(x_{\mathrm{dd}}-x_{l}\right)\,\left(\frac{\psi _{\mathrm{1d},\mathrm{SG},D,1}\,\left(x_{\mathrm{dd}}-x_{\mathrm{ddd}}\right)}{x_{\mathrm{dd}}-x_{l}}-\psi _{d,\mathrm{SG},D,1}+\frac{\psi _{\mathrm{fd},\mathrm{SG},D,1}\,\left(x_{\mathrm{ddd}}-x_{l}\right)}{x_{\mathrm{dd}}-x_{l}}\right)}{x_{\mathrm{ddd}}}\right)}{{\left(x_{\mathrm{dd}}-x_{l}\right)}^2}\right)}{T_{\mathrm{dd}}}$
      | Automatically generated on 2025-10-31 19:23:12 .
  State_E_fd_SG_D_1_9c11e : Inport
  State_psi_fd_SG_D_1_89de8 : Inport  Port=2
  State_psi_1d_SG_D_1_80808 : Inport  Port=3
  State_psi_fd_SG_D_1_3f013 : Inport  Port=4
  State_psi_1d_SG_D_1_e7af2 : Inport  Port=5
  State_psi_d_SG_D_1_6490f : Inport  Port=6
  State_psi_fd_SG_D_1_23553 : Inport  Port=7
  State_psi_1d_SG_D_1_8dc8e : Inport  Port=8
  State_psi_d_SG_D_1_0357b : Inport  Port=9
  State_psi_fd_SG_D_1_d4d2a : Inport  Port=10
  Add_4ecab : Sum
  Add_db39a : Sum
  Constant_-1_3569a : Constant  Value=-1
  Constant_-1_db80d : Constant  Value=-1
  Constant_-1_e6b07 : Constant  Value=-1
  Constant_2.0_4cfad : Constant  Value=2.0
  Constant_T_dd_c9818 : Constant  Value=T_dd
  Constant_x_d_80cf6 : Constant  Value=x_d
  Constant_x_dd_148b7 : Constant  Value=x_dd
  Constant_x_dd_2a1ab : Constant  Value=x_dd
  Constant_x_dd_40312 : Constant  Value=x_dd
  Constant_x_dd_41f85 : Constant  Value=x_dd
  Constant_x_dd_597a4 : Constant  Value=x_dd
  Constant_x_dd_7163f : Constant  Value=x_dd
  Constant_x_dd_920c9 : Constant  Value=x_dd
  Constant_x_dd_a8264 : Constant  Value=x_dd
  Constant_x_dd_e2968 : Constant  Value=x_dd
  Constant_x_dd_e84ce : Constant  Value=x_dd
  Constant_x_ddd_2bf3a : Constant  Value=x_ddd
  Constant_x_ddd_3597c : Constant  Value=x_ddd
  Constant_x_ddd_42fd2 : Constant  Value=x_ddd
  Constant_x_ddd_4430b : Constant  Value=x_ddd
  Constant_x_ddd_44430 : Constant  Value=x_ddd
  Constant_x_ddd_bfcf1 : Constant  Value=x_ddd
  Constant_x_ddd_e3936 : Constant  Value=x_ddd
  Constant_x_l_0e026 : Constant  Value=x_l
  Constant_x_l_456a2 : Constant  Value=x_l
  Constant_x_l_76080 : Constant  Value=x_l
  Constant_x_l_783cf : Constant  Value=x_l
  Constant_x_l_9ccfd : Constant  Value=x_l
  Constant_x_l_b1484 : Constant  Value=x_l
  Constant_x_l_b4575 : Constant  Value=x_l
  Constant_x_l_e2858 : Constant  Value=x_l
  Divide_2821e : Product  Inputs=*/
  Divide_2d16f : Product  Inputs=*/
  Divide_75069 : Product  Inputs=*/
  Divide_86d86 : Product  Inputs=*/
  Divide_b16f4 : Product  Inputs=*/
  Divide_b59cf : Product  Inputs=*/
  Divide_c3aa2 : Product  Inputs=*/
  Divide_eafbc : Product  Inputs=*/
  Power_3027c : Math  Operator=pow
  Product_07c28 : Product
  Product_17f03 : Product
  Product_47dc5 : Product
  Product_4a915 : Product
  Product_7bfc8 : Product
  Product_8361c : Product
  Product_bbc17 : Product
  Product_c64a0 : Product
  Product_c66dd : Product
  Product_d0efb : Product
  Subtract_21bea : Sum  Inputs=+-
  Subtract_30bc9 : Sum  Inputs=+-
  Subtract_329ed : Sum  Inputs=+-
  Subtract_3a145 : Sum  Inputs=+-
  Subtract_49633 : Sum  Inputs=+-
  Subtract_4a569 : Sum  Inputs=+-
  Subtract_53079 : Sum  Inputs=+-
  Subtract_60de9 : Sum  Inputs=+-
  Subtract_651e7 : Sum  Inputs=+-
  Subtract_7138f : Sum  Inputs=+-
  Subtract_7371b : Sum  Inputs=+-
  Subtract_795a6 : Sum  Inputs=+-
  Subtract_986d8 : Sum  Inputs=+-
  Subtract_9b736 : Sum  Inputs=+-
  Subtract_9ee56 : Sum  Inputs=+-
  Subtract_cc9f3 : Sum  Inputs=+-
  Subtract_cd0a4 : Sum  Inputs=+-
  Subtract_ef77d : Sum  Inputs=+-
  Subtract_f543c : Sum  Inputs=+-
  Blockout_d_psi_fd_SG_D_1_20036 : Outport
  wires:
  State_psi_d_SG_D_1_6490f/1 -> Add_4ecab/2
  Constant_x_dd_e84ce/1 -> Subtract_9ee56/1
  Product_47dc5/1 -> Divide_c3aa2/1
  Subtract_4a569/1 -> Product_47dc5/2
  Subtract_53079/1 -> Product_8361c/2
  Product_17f03/1 -> Product_47dc5/1
  Constant_x_dd_920c9/1 -> Subtract_4a569/1
  Constant_x_l_76080/1 -> Subtract_986d8/2
  Constant_-1_db80d/1 -> Product_17f03/1
  Subtract_986d8/1 -> Product_8361c/1
  Constant_x_l_e2858/1 -> Subtract_9ee56/2
  Constant_x_ddd_2bf3a/1 -> Subtract_4a569/2
  State_psi_1d_SG_D_1_e7af2/1 -> Product_17f03/2
  Constant_x_ddd_4430b/1 -> Subtract_651e7/1
  Constant_x_l_783cf/1 -> Subtract_651e7/2
  State_E_fd_SG_D_1_9c11e/1 -> Subtract_cc9f3/1
  Divide_c3aa2/1 -> Add_4ecab/1
  Subtract_9ee56/1 -> Divide_c3aa2/2
  State_psi_fd_SG_D_1_23553/1 -> Product_bbc17/1
  Constant_x_ddd_3597c/1 -> Divide_86d86/2
  Subtract_651e7/1 -> Product_bbc17/2
  Constant_x_dd_41f85/1 -> Subtract_3a145/1
  Constant_x_dd_a8264/1 -> Subtract_f543c/1
  State_psi_fd_SG_D_1_89de8/1 -> Subtract_cc9f3/2
  Constant_x_l_456a2/1 -> Subtract_3a145/2
  Product_bbc17/1 -> Divide_b16f4/1
  Constant_-1_3569a/1 -> Product_7bfc8/1
  Subtract_3a145/1 -> Divide_b16f4/2
  Constant_x_dd_e2968/1 -> Subtract_986d8/1
  Add_4ecab/1 -> Subtract_53079/1
  Constant_x_l_0e026/1 -> Subtract_f543c/2
  Divide_b16f4/1 -> Subtract_53079/2
  Divide_2d16f/1 -> Subtract_60de9/1
  Constant_-1_e6b07/1 -> Product_4a915/1
  State_psi_1d_SG_D_1_8dc8e/1 -> Product_4a915/2
  Constant_x_dd_7163f/1 -> Subtract_21bea/1
  Subtract_329ed/1 -> Product_7bfc8/2
  Constant_x_ddd_bfcf1/1 -> Subtract_21bea/2
  Product_4a915/1 -> Product_d0efb/1
  Constant_2.0_4cfad/1 -> Power_3027c/2
  Product_d0efb/1 -> Divide_75069/1
  Subtract_60de9/1 -> Product_c66dd/2
  Subtract_21bea/1 -> Product_d0efb/2
  State_psi_d_SG_D_1_0357b/1 -> Add_db39a/2
  Constant_x_dd_2a1ab/1 -> Subtract_30bc9/1
  Constant_x_l_9ccfd/1 -> Subtract_30bc9/2
  Constant_x_dd_597a4/1 -> Subtract_329ed/1
  Divide_86d86/1 -> Subtract_49633/2
  Constant_x_ddd_44430/1 -> Subtract_795a6/1
  Constant_x_ddd_42fd2/1 -> Subtract_329ed/2
  Constant_x_l_b1484/1 -> Subtract_795a6/2
  Subtract_795a6/1 -> Product_07c28/2
  State_psi_1d_SG_D_1_80808/1 -> Subtract_9b736/1
  Product_07c28/1 -> Divide_2821e/1
  State_psi_fd_SG_D_1_3f013/1 -> Subtract_9b736/2
  State_psi_fd_SG_D_1_d4d2a/1 -> Product_07c28/1
  Product_8361c/1 -> Divide_86d86/1
  Divide_75069/1 -> Add_db39a/1
  Subtract_30bc9/1 -> Divide_75069/2
  Constant_x_dd_148b7/1 -> Subtract_cd0a4/1
  Constant_x_l_b4575/1 -> Subtract_cd0a4/2
  Divide_2821e/1 -> Subtract_7371b/2
  Subtract_9b736/1 -> Subtract_49633/1
  Subtract_cd0a4/1 -> Divide_2821e/2
  Subtract_49633/1 -> Product_c64a0/2
  Product_7bfc8/1 -> Product_c64a0/1
  Subtract_f543c/1 -> Power_3027c/1
  Add_db39a/1 -> Subtract_7371b/1
  Product_c64a0/1 -> Divide_2d16f/1
  Power_3027c/1 -> Divide_2d16f/2
  Subtract_7371b/1 -> Divide_eafbc/1
  Constant_x_ddd_e3936/1 -> Divide_eafbc/2
  Constant_x_d_80cf6/1 -> Subtract_ef77d/1
  Constant_x_dd_40312/1 -> Subtract_ef77d/2
  Divide_eafbc/1 -> Subtract_60de9/2
  Subtract_ef77d/1 -> Product_c66dd/1
  Subtract_cc9f3/1 -> Subtract_7138f/1
  Product_c66dd/1 -> Subtract_7138f/2
  Subtract_7138f/1 -> Divide_b59cf/1
  Constant_T_dd_c9818/1 -> Divide_b59cf/2
  Divide_b59cf/1 -> Blockout_d_psi_fd_SG_D_1_20036/1

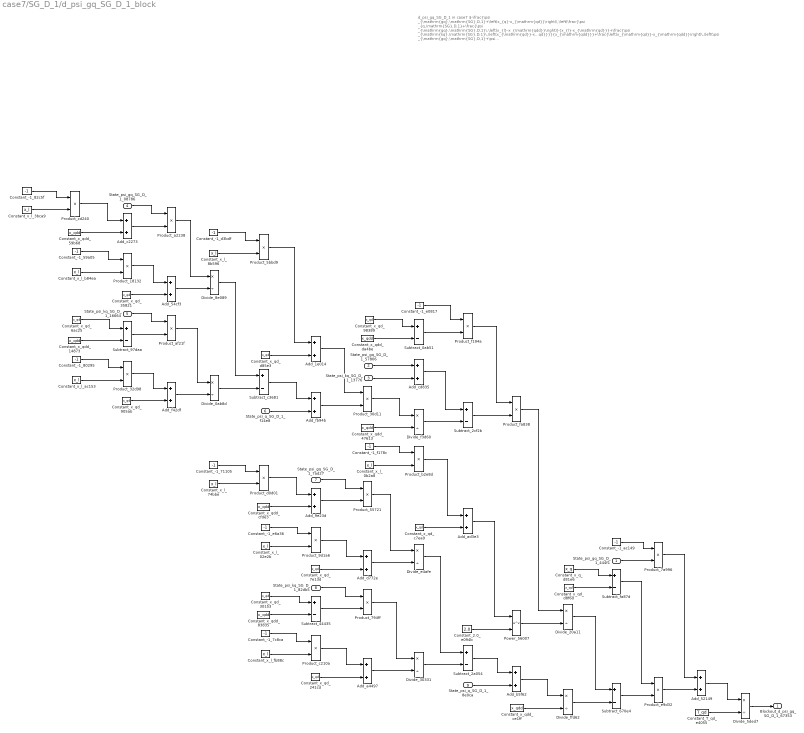
== system case7/SG_D_1/d_psi_gq_SG_D_1_block ==
  note: d_psi_gq_SG_D_1 in case7
      | $-\frac{\psi _{\mathrm{gq},\mathrm{SG},D,1}+\left(x_{q}-x_{\mathrm{qd}}\right)\,\left(\frac{\psi _{q,\mathrm{SG},D,1}+\frac{\psi _{\mathrm{gq},\mathrm{SG},D,1}\,\left(x_{l}-x_{\mathrm{qdd}}\right)}{x_{l}-x_{\mathrm{qd}}}+\frac{\psi _{\mathrm{kq},\mathrm{SG},D,1}\,\left(x_{\mathrm{qd}}-x_{\mathrm{qdd}}\right)}{x_{l}-x_{\mathrm{qd}}}}{x_{\mathrm{qdd}}}+\frac{\left(x_{\mathrm{qd}}-x_{\mathrm{qdd}}\right)\,\left(\psi _{\mathrm{gq},\mathrm{SG},D,1}+\psi _{\mathrm{kq},\mathrm{SG},D,1}+\frac{\left(x_{l}-x_{\mathrm{qd}}\right)\,\left(\psi _{q,\mathrm{SG},D,1}+\frac{\psi _{\mathrm{gq},\mathrm{SG},D,1}\,\left(x_{l}-x_{\mathrm{qdd}}\right)}{x_{l}-x_{\mathrm{qd}}}+\frac{\psi _{\mathrm{kq},\mathrm{SG},D,1}\,\left(x_{\mathrm{qd}}-x_{\mathrm{qdd}}\right)}{x_{l}-x_{\mathrm{qd}}}\right)}{x_{\mathrm{qdd}}}\right)}{{\left(x_{l}-x_{\mathrm{qd}}\right)}^2}\right)}{T_{\mathrm{qd}}}$
      | Automatically generated on 2025-10-31 19:23:21 .
  State_psi_gq_SG_D_1_444f1 : Inport
  State_psi_gq_SG_D_1_57806 : Inport  Port=2
  State_psi_kq_SG_D_1_13776 : Inport  Port=3
  State_psi_gq_SG_D_1_08786 : Inport  Port=4
  State_psi_kq_SG_D_1_16664 : Inport  Port=5
  State_psi_q_SG_D_1_f14e8 : Inport  Port=6
  State_psi_gq_SG_D_1_7ad27 : Inport  Port=7
  State_psi_kq_SG_D_1_82db5 : Inport  Port=8
  State_psi_q_SG_D_1_8e0ca : Inport  Port=9
  Add_1e014 : Sum
  Add_52149 : Sum
  Add_54cf3 : Sum
  Add_9e23d : Sum
  Add_a4497 : Sum
  Add_ad3e3 : Sum
  Add_b5f62 : Sum
  Add_c2273 : Sum
  Add_cd835 : Sum
  Add_d772e : Sum
  Add_f42df : Sum
  Add_fb94b : Sum
  Constant_-1_59a05 : Constant  Value=-1
  Constant_-1_71105 : Constant  Value=-1
  Constant_-1_7c8ca : Constant  Value=-1
  Constant_-1_80295 : Constant  Value=-1
  Constant_-1_82c5f : Constant  Value=-1
  Constant_-1_ac149 : Constant  Value=-1
  Constant_-1_d3bdf : Constant  Value=-1
  Constant_-1_e0817 : Constant  Value=-1
  Constant_-1_e6a36 : Constant  Value=-1
  Constant_-1_f178c : Constant  Value=-1
  Constant_2.0_e094b : Constant  Value=2.0
  Constant_T_qd_e4055 : Constant  Value=T_qd
  Constant_x_l_02e2b : Constant  Value=x_l
  Constant_x_l_0b2a8 : Constant  Value=x_l
  Constant_x_l_3bca9 : Constant  Value=x_l
  Constant_x_l_74bbe : Constant  Value=x_l
  Constant_x_l_8b596 : Constant  Value=x_l
  Constant_x_l_ac153 : Constant  Value=x_l
  Constant_x_l_b84ea : Constant  Value=x_l
  Constant_x_l_fb88c : Constant  Value=x_l
  Constant_x_q_d81e6 : Constant  Value=x_q
  Constant_x_qd_241cd : Constant  Value=x_qd
  Constant_x_qd_30153 : Constant  Value=x_qd
  Constant_x_qd_35821 : Constant  Value=x_qd
  Constant_x_qd_6ac25 : Constant  Value=x_qd
  Constant_x_qd_7e13d : Constant  Value=x_qd
  Constant_x_qd_905ab : Constant  Value=x_qd
  Constant_x_qd_98389 : Constant  Value=x_qd
  Constant_x_qd_c7ea9 : Constant  Value=x_qd
  Constant_x_qd_d85e3 : Constant  Value=x_qd
  Constant_x_qd_d8f6d : Constant  Value=x_qd
  Constant_x_qdd_14873 : Constant  Value=x_qdd
  Constant_x_qdd_47613 : Constant  Value=x_qdd
  Constant_x_qdd_59b68 : Constant  Value=x_qdd
  Constant_x_qdd_83835 : Constant  Value=x_qdd
  Constant_x_qdd_ce1ff : Constant  Value=x_qdd
  Constant_x_qdd_cfde3 : Constant  Value=x_qdd
  Constant_x_qdd_da4be : Constant  Value=x_qdd
  Divide_0ab8d : Product  Inputs=*/
  Divide_20a11 : Product  Inputs=*/
  Divide_30331 : Product  Inputs=*/
  Divide_5ded7 : Product  Inputs=*/
  Divide_8e089 : Product  Inputs=*/
  Divide_e4afe : Product  Inputs=*/
  Divide_f3d60 : Product  Inputs=*/
  Divide_ffd62 : Product  Inputs=*/
  Power_56007 : Math  Operator=pow
  Product_18132 : Product
  Product_30d11 : Product
  Product_32d98 : Product
  Product_55721 : Product
  Product_5bbd9 : Product
  Product_794ff : Product
  Product_7a996 : Product
  Product_9d1a6 : Product
  Product_a2238 : Product
  Product_af21f : Product
  Product_b2e8d : Product
  Product_c210a : Product
  Product_cd240 : Product
  Product_d0d01 : Product
  Product_e9d32 : Product
  Product_f194a : Product
  Product_fa838 : Product
  Subtract_0ab51 : Sum  Inputs=+-
  Subtract_2a054 : Sum  Inputs=+-
  Subtract_2cf2b : Sum  Inputs=+-
  Subtract_44435 : Sum  Inputs=+-
  Subtract_670e4 : Sum  Inputs=+-
  Subtract_97daa : Sum  Inputs=+-
  Subtract_c3681 : Sum  Inputs=+-
  Subtract_fa87d : Sum  Inputs=+-
  Blockout_d_psi_gq_SG_D_1_67353 : Outport
  wires:
  State_psi_gq_SG_D_1_08786/1 -> Product_a2238/1
  Constant_-1_59a05/1 -> Product_18132/1
  Divide_8e089/1 -> Subtract_c3681/1
  Add_54cf3/1 -> Divide_8e089/2
  Product_cd240/1 -> Add_c2273/1
  Constant_x_qd_d85e3/1 -> Add_1e014/2
  Constant_-1_82c5f/1 -> Product_cd240/1
  Constant_x_qdd_59b68/1 -> Add_c2273/2
  Constant_x_l_b84ea/1 -> Product_18132/2
  Constant_x_l_3bca9/1 -> Product_cd240/2
  Constant_-1_80295/1 -> Product_32d98/1
  Constant_x_qd_6ac25/1 -> Subtract_97daa/1
  Constant_x_qdd_47613/1 -> Divide_f3d60/2
  Constant_x_l_ac153/1 -> Product_32d98/2
  Constant_x_qdd_14873/1 -> Subtract_97daa/2
  Subtract_c3681/1 -> Add_fb94b/1
  Add_c2273/1 -> Product_a2238/2
  Product_a2238/1 -> Divide_8e089/1
  Product_18132/1 -> Add_54cf3/1
  Constant_x_qd_35821/1 -> Add_54cf3/2
  State_psi_kq_SG_D_1_16664/1 -> Product_af21f/1
  Product_32d98/1 -> Add_f42df/1
  Subtract_97daa/1 -> Product_af21f/2
  Constant_x_qd_905ab/1 -> Add_f42df/2
  Product_af21f/1 -> Divide_0ab8d/1
  Add_f42df/1 -> Divide_0ab8d/2
  Constant_-1_e0817/1 -> Product_f194a/1
  Constant_-1_d3bdf/1 -> Product_5bbd9/1
  Add_d772e/1 -> Divide_e4afe/2
  Product_c210a/1 -> Add_a4497/1
  Subtract_44435/1 -> Product_794ff/2
  Constant_x_l_8b596/1 -> Product_5bbd9/2
  Divide_0ab8d/1 -> Subtract_c3681/2
  Subtract_fa87d/1 -> Product_e9d32/1
  Constant_-1_f178c/1 -> Product_b2e8d/1
  Constant_-1_71105/1 -> Product_d0d01/1
  Constant_x_l_0b2a8/1 -> Product_b2e8d/2
  Constant_x_l_74bbe/1 -> Product_d0d01/2
  Constant_x_qd_7e13d/1 -> Add_d772e/2
  Product_5bbd9/1 -> Add_1e014/1
  State_psi_q_SG_D_1_f14e8/1 -> Add_fb94b/2
  Product_d0d01/1 -> Add_9e23d/1
  Constant_x_qdd_cfde3/1 -> Add_9e23d/2
  Constant_-1_e6a36/1 -> Product_9d1a6/1
  Constant_x_qd_241cd/1 -> Add_a4497/2
  Add_1e014/1 -> Product_30d11/1
  Constant_x_l_02e2b/1 -> Product_9d1a6/2
  Constant_-1_7c8ca/1 -> Product_c210a/1
  Constant_x_qd_30153/1 -> Subtract_44435/1
  Product_30d11/1 -> Divide_f3d60/1
  Constant_x_l_fb88c/1 -> Product_c210a/2
  Divide_20a11/1 -> Subtract_670e4/1
  Constant_x_qdd_83835/1 -> Subtract_44435/2
  Add_fb94b/1 -> Product_30d11/2
  State_psi_gq_SG_D_1_7ad27/1 -> Product_55721/1
  Add_9e23d/1 -> Product_55721/2
  Product_9d1a6/1 -> Add_d772e/1
  State_psi_kq_SG_D_1_82db5/1 -> Product_794ff/1
  Add_a4497/1 -> Divide_30331/2
  State_psi_gq_SG_D_1_57806/1 -> Add_cd835/1
  Constant_x_qd_98389/1 -> Subtract_0ab51/1
  Constant_x_qdd_da4be/1 -> Subtract_0ab51/2
  Product_794ff/1 -> Divide_30331/1
  State_psi_kq_SG_D_1_13776/1 -> Add_cd835/2
  Product_55721/1 -> Divide_e4afe/1
  Subtract_0ab51/1 -> Product_f194a/2
  Add_cd835/1 -> Subtract_2cf2b/1
  Divide_f3d60/1 -> Subtract_2cf2b/2
  Product_b2e8d/1 -> Add_ad3e3/1
  Constant_x_qd_c7ea9/1 -> Add_ad3e3/2
  Divide_e4afe/1 -> Subtract_2a054/1
  Divide_30331/1 -> Subtract_2a054/2
  Product_f194a/1 -> Product_fa838/1
  Subtract_2cf2b/1 -> Product_fa838/2
  Add_ad3e3/1 -> Power_56007/1
  Constant_2.0_e094b/1 -> Power_56007/2
  Subtract_2a054/1 -> Add_b5f62/1
  State_psi_q_SG_D_1_8e0ca/1 -> Add_b5f62/2
  Product_fa838/1 -> Divide_20a11/1
  Power_56007/1 -> Divide_20a11/2
  Add_b5f62/1 -> Divide_ffd62/1
  Constant_x_qdd_ce1ff/1 -> Divide_ffd62/2
  Constant_x_q_d81e6/1 -> Subtract_fa87d/1
  Constant_x_qd_d8f6d/1 -> Subtract_fa87d/2
  Divide_ffd62/1 -> Subtract_670e4/2
  Constant_-1_ac149/1 -> Product_7a996/1
  State_psi_gq_SG_D_1_444f1/1 -> Product_7a996/2
  Subtract_670e4/1 -> Product_e9d32/2
  Product_7a996/1 -> Add_52149/1
  Product_e9d32/1 -> Add_52149/2
  Add_52149/1 -> Divide_5ded7/1
  Constant_T_qd_e4055/1 -> Divide_5ded7/2
  Divide_5ded7/1 -> Blockout_d_psi_gq_SG_D_1_67353/1
